simulink model "Coords_Model_1_alt_variation"  (R2019b)
settings: Solver=ode45  StartTime=0.0  StopTime=250  MaxStep=0.02  RelTol=1e-5  AbsTol=1e-7
undefined symbols (not defined in the file): f, ft, m, s
libraries: simulink x6, aerolibutil x2, aerolibconvert2 x2, shared6dof x1, vrlib x1, aerolibconvert x1, dspsnks4 x1, dspvision x1
Description:
  | Six Degree of Freedom Motion Platform
  | 
  | This model shows how to connect an Aerospace Blockset(TM) six degree of freedom
  | equation of motion block.
settings Model: SimulationMode=accelerator  ExtModeTrigMode=oneshot  ExtModeArmWhenConnect=off  ExtModeAutoUpdateStatusClock=off  Creator=The MathWorks, Inc.  LastModifiedBy=Admin
settings SolverCC: AutoScaleAbsTol=off
settings DataIOCC: SaveFormat=Array  SaveOutput=off  ReturnWorkspaceOutputs=off
settings OptimizationCC: DefaultParameterBehavior=Inlined  InlineInvariantSignals=on  ExpressionDepthLimit=2147483647  InitFltsAndDblsToZero=on  EfficientFloat2IntCast=on  LifeSpan=inf
settings DebuggingCC: SaveWithParameterizedLinksMsg=none  MultiTaskCondExecSysMsg=none  SigSpecEnsureSampleTimeMsg=none  FcnCallInpInsideContextMsg=warning  UniqueDataStoreMsg=error  StateNameClashWarn=warning  StrictBusMsg=ErrorOnBusTreatedAsVector  SFUnexpectedBacktrackingDiag=warning  SFNoUnconditionalDefaultTransitionDiag=warning  SFExecutionAtInitializationDiag=none  ArithmeticOperatorsInVariantConditions=warning
settings HardwareCC: ProdBitPerPointer=32  ProdLargestAtomicFloat=None  ProdIntDivRoundTo=Undefined  ProdEndianess=Unspecified  ProdWordSize=32  ProdHWDeviceType=32-bit Generic  TargetUnknown=on
settings ModelReferenceCC: PropagateSignalLabelsOutOfModel=off
settings SFSimCC: SimUseLocalCustomCode=off  CustomCodeUndefinedFunction=UseInterfaceOnly
settings RTWCC: TemplateMakefile=grt_vc.tmf  RTWUseLocalCustomCode=off
settings CodeAppCC: StateflowObjectComments=on
settings GRTTargetCC: TargetFcnLib=ansi_tfl_tmw.mat  TargetLangStandard=C89/C90 (ANSI)  GeneratePreprocessorConditionals=Disable all  CombineOutputUpdateFcns=off  GRTInterface=on
settings ConfigComp: CovMetricSettings=d  CovHtmlReporting=on  CovSaveCumulativeToWorkspaceVar=on  CovSaveSingleToWorkspaceVar=on  CovExternalEMLEnable=off

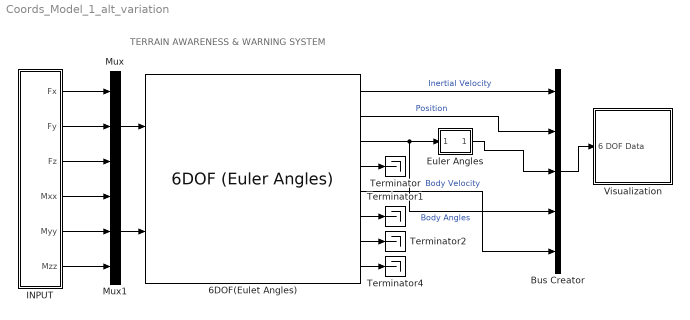
== system Coords_Model_1_alt_variation ==
  note: TERRAIN AWARENESS & WARNING SYSTEM
  "6DOF(Eulet Angles) " : shared6dof/6DOF (Euler Angles)  units=Metric (MKS)  mtype=Fixed  rep=Euler Angles  xme_0=[8500 0 -850]  Vm_0=[0 -75 0]  eul_0=[-0.05 0.1 -0.1]  pm_0=[0 0 0]  mass_0=1.0  mass_e=0.5  mass_f=2.0  inertia=eye(3)  inertia_e=eye(3)  inertia_f=2*eye(3)  k_quat=1.0  vre_flag=on  abi_flag=off  aMode=0  xme_statename=''  Vm_statename=''  eul_statename=''  quat_statename=''  pm_statename=''  mass_statename=''
      settings: SourceProductBaseCode=AE
  Bus Creator : BusCreator  Inputs=5
  Euler Angles : Subsystem
  INPUT : Subsystem
  Mux : Mux  Inputs=3
  Mux1 : Mux  Inputs=3
  Terminator{,1..2,4} (4 alike) : Terminator
  Visualization : Subsystem
  wires:
  Mux1/1 -> "6DOF(Eulet Angles) "/2
  Mux/1 -> "6DOF(Eulet Angles) "/1
  "6DOF(Eulet Angles) "/1 -> Bus Creator/1  "Inertial Velocity"
  "6DOF(Eulet Angles) "/2 -> Bus Creator/2  "Position"
  "6DOF(Eulet Angles) "/3 -> Bus Creator/4, Euler Angles/1(body angles)  "Body Angles"
  "6DOF(Eulet Angles) "/5 -> Bus Creator/5  "Body Velocity"
  Bus Creator/1 -> Visualization/1(6 DOF Data)
  INPUT/1(Fx) -> Mux/1
  INPUT/2(Fy) -> Mux/2
  INPUT/3(Fz) -> Mux/3
  INPUT/4(Mxx) -> Mux1/1
  INPUT/5(Myy) -> Mux1/2
  INPUT/6(Mzz) -> Mux1/3
  Euler Angles/1(euler angles) -> Bus Creator/3
  "6DOF(Eulet Angles) "/4 -> Terminator/1
  "6DOF(Eulet Angles) "/6 -> Terminator1/1
  "6DOF(Eulet Angles) "/7 -> Terminator2/1
  "6DOF(Eulet Angles) "/8 -> Terminator4/1

== system Coords_Model_1_alt_variation/Euler Angles ==
  body angles : Inport
  Bus Creator1 : BusCreator  Inputs=3
  Demux : Demux  Outputs=3
  euler angles : Outport
  wires:
  body angles/1 -> Demux/1
  Bus Creator1/1 -> euler angles/1  "euler angles"
  Demux/1 -> Bus Creator1/1  "psi"
  Demux/2 -> Bus Creator1/2  "theta"
  Demux/3 -> Bus Creator1/3  "phi"

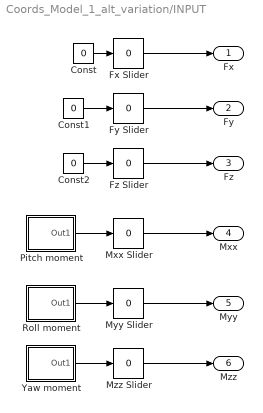
== system Coords_Model_1_alt_variation/INPUT ==
  Const : Constant  Value=0
  Const1 : Constant  Value=0
  Const2 : Constant  Value=0
  Fx Slider : simulink/Math Operations/Slider Gain  gain=0  low=-1  high=1
  Fy Slider : simulink/Math Operations/Slider Gain  gain=0  low=-1  high=1
  Fz Slider : simulink/Math Operations/Slider Gain  gain=0  low=-1  high=1
  Mxx Slider : simulink/Math Operations/Slider Gain  gain=0  low=-5  high=10
  Myy Slider : simulink/Math Operations/Slider Gain  gain=0  low=-10  high=10
  Mzz Slider : simulink/Math Operations/Slider Gain  gain=0  low=-1  high=1
  Pitch moment : Subsystem  mask(timed input){t=[0 3 3 4 4 5 5  7.5 7.5 8.5 8.5 9.5 9.5 10], u=[0 0  1 1 -1 -1.005 0 0 -1 -1 1 1 0 0]*3.138/2}
      mask prompts: t "time values:"; u "input values"
      mask Display: plot(t,u)
  Roll moment : Subsystem  mask(timed input){t=[0 1 1 2 2  10], u=[1 1 -1 -.998  0 0]*3.144/2}
      mask prompts: t "time values:"; u "input values"
      mask Display: plot(t,u)
  Yaw moment : Subsystem  mask(timed input){t=[0 6 6 7 7 8 8 10], u=[0 0  -1 -1 1 1 0 0]*3.1/2}
      mask prompts: t "time values:"; u "input values"
      mask Display: plot(t,u)
  Fx : Outport
  Fy : Outport  Port=2
  Fz : Outport  Port=3
  Mxx : Outport  Port=4
  Myy : Outport  Port=5
  Mzz : Outport  Port=6
  wires:
  Roll moment/1(Out1) -> Myy Slider/1
  Yaw moment/1(Out1) -> Mzz Slider/1
  Const2/1 -> Fz Slider/1
  Const/1 -> Fx Slider/1
  Pitch moment/1(Out1) -> Mxx Slider/1
  Const1/1 -> Fy Slider/1
  Fy Slider/1 -> Fy/1
  Mxx Slider/1 -> Mxx/1
  Myy Slider/1 -> Myy/1
  Fz Slider/1 -> Fz/1
  Fx Slider/1 -> Fx/1
  Mzz Slider/1 -> Mzz/1

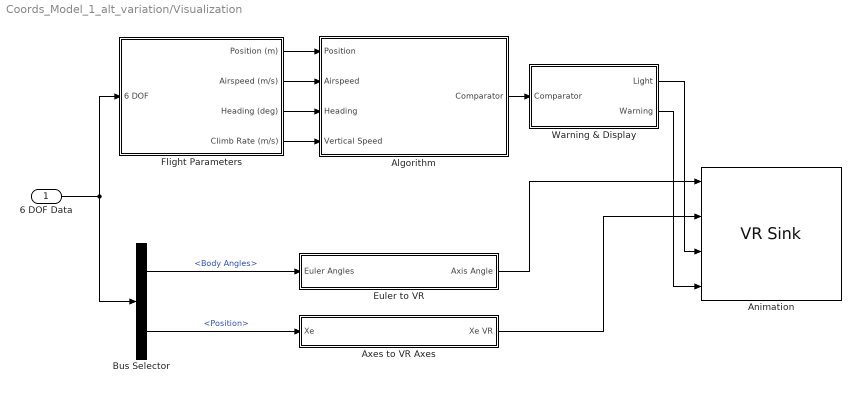
== system Coords_Model_1_alt_variation/Visualization ==
  6 DOF Data : Inport
  Algorithm : Subsystem
  Animation : vrlib/VR Sink  InstantiateOnLoad=on  SampleTime=0.1  ViewEnable=on  RemoteChange=off  RemoteView=off  FieldsWritten=Plane.rotation.4.1.1.double#Plane.translation.3.1.1.double#Light.diffuseColor.3.1.1.double#Warning.string.1.-1.1.char  WorldFileName=Coods_Updated.wrl  WorldDescription=VR Plane Take-Off with HUD Text  AutoView=off  VideoDimensions=[]  AllowVariableSize=off
      settings: SourceProductName=Simulink
  Axes to VR Axes : Subsystem
  Bus Selector : BusSelector  OutputSignals=Body Angles,Position
  Euler to VR : Subsystem
  "Flight Parameters " : Subsystem
  Warning & Display : Subsystem
  wires:
  6 DOF Data/1 -> Bus Selector/1, "Flight Parameters "/1("6 DOF ")
  Bus Selector/2 -> Axes to VR Axes/1(Xe)  "<Position>"
  Bus Selector/1 -> Euler to VR/1(Euler Angles)  "<Body Angles>"
  Algorithm/1(Comparator) -> Warning & Display/1(Comparator)
  "Flight Parameters "/1(Position (m)) -> Algorithm/1(Position)
  "Flight Parameters "/2(Airspeed (m/s)) -> Algorithm/2(Airspeed)
  "Flight Parameters "/3(Heading (deg)) -> Algorithm/3(Heading)
  Warning & Display/1(Light) -> Animation/3
  Warning & Display/2(Warning) -> Animation/4
  Euler to VR/1(Axis Angle) -> Animation/1
  Axes to VR Axes/1(Xe VR) -> Animation/2
  "Flight Parameters "/4(Climb Rate (m/s)) -> Algorithm/4(Vertical Speed)

== system Coords_Model_1_alt_variation/INPUT/Pitch moment ==
  From Workspace : FromWorkspace  VariableName=[t',u']  SampleTime=0
  Out1 : Outport  VectorParamsAs1DForOutWhenUnconnected=off
  wires:
  From Workspace/1 -> Out1/1

== system Coords_Model_1_alt_variation/INPUT/Roll moment ==
  From Workspace : FromWorkspace  VariableName=[t',u']  SampleTime=0
  Out1 : Outport  VectorParamsAs1DForOutWhenUnconnected=off
  wires:
  From Workspace/1 -> Out1/1

== system Coords_Model_1_alt_variation/INPUT/Yaw moment ==
  From Workspace : FromWorkspace  VariableName=[t',u']  SampleTime=0
  Out1 : Outport  VectorParamsAs1DForOutWhenUnconnected=off
  wires:
  From Workspace/1 -> Out1/1

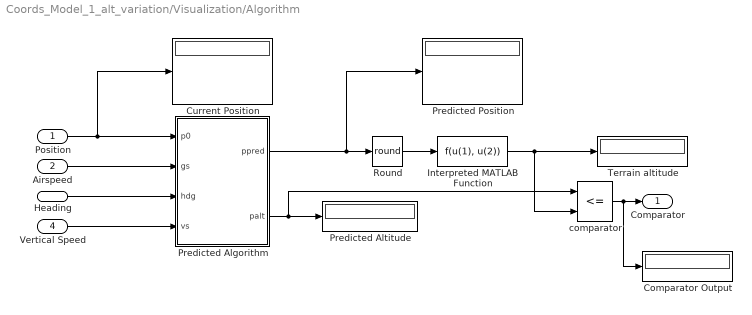
== system Coords_Model_1_alt_variation/Visualization/Algorithm ==
  Position : Inport
  Airspeed : Inport  Port=2
  Heading : Inport  Port=3
  Vertical Speed : Inport  Port=4
  Comparator Output : Display
  Current Position : Display
  Interpreted MATLAB Function : MATLABFcn  MATLABFcn=f(u(1), u(2))
      mask init:
      | load('interpo.mat')
  Predicted Algorithm : MATLAB Function  TreatAsAtomicUnit=on
  Predicted Altitude : Display
      settings: Format=bank
  Predicted Position : Display
  Round : Rounding  Operator=round
  Terrain altitude : Display
  comparator : RelationalOperator  Operator=<=  OutDataTypeStr=boolean  RndMeth=Simplest
  Comparator : Outport
  wires:
  Heading/1 -> Predicted Algorithm/3(hdg)
  Round/1 -> Interpreted MATLAB Function/1
  Interpreted MATLAB Function/1 -> Terrain altitude/1, comparator/2
  Position/1 -> Current Position/1, Predicted Algorithm/1(p0)
  Predicted Algorithm/2(palt) -> Predicted Altitude/1, comparator/1
  Airspeed/1 -> Predicted Algorithm/2(gs)
  comparator/1 -> Comparator Output/1, Comparator/1
  Predicted Algorithm/1(ppred) -> Predicted Position/1, Round/1
  Vertical Speed/1 -> Predicted Algorithm/4(vs)

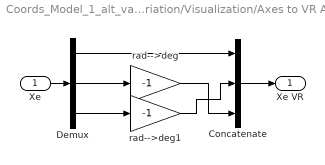
== system Coords_Model_1_alt_variation/Visualization/Axes to VR Axes ==
  Xe : Inport
  Concatenate : Concatenate  NumInputs=3
  Demux : Demux  Outputs=3
  rad-->deg : Gain  Gain=-1  SaturateOnIntegerOverflow=on  OutDataTypeStr=Inherit: Same as input  ParamDataTypeStr=Inherit: Same as input
  rad-->deg1 : Gain  Gain=-1  SaturateOnIntegerOverflow=on  OutDataTypeStr=Inherit: Same as input  ParamDataTypeStr=Inherit: Same as input
  Xe VR : Outport  VectorParamsAs1DForOutWhenUnconnected=off
  wires:
  Xe/1 -> Demux/1
  Demux/1 -> Concatenate/1
  Demux/2 -> rad-->deg/1
  Demux/3 -> rad-->deg1/1
  Concatenate/1 -> Xe VR/1
  rad-->deg1/1 -> Concatenate/2
  rad-->deg/1 -> Concatenate/3

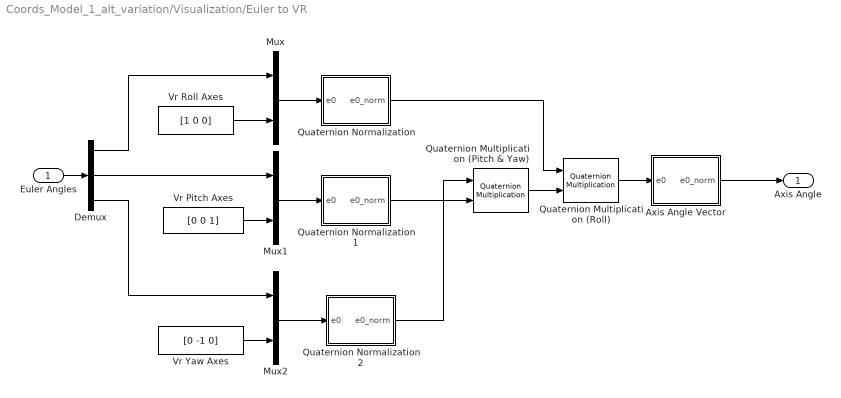
== system Coords_Model_1_alt_variation/Visualization/Euler to VR ==
  Euler Angles : Inport
  Axis Angle Vector : Subsystem
  Demux : Demux  Outputs=3
  Mux : Mux  Inputs=2
  Mux1 : Mux  Inputs=2
  Mux2 : Mux  Inputs=2
  Quaternion Multiplication (Pitch & Yaw) : aerolibutil/Quaternion Multiplication
  Quaternion Multiplication (Roll) : aerolibutil/Quaternion Multiplication
  Quaternion Normalization : Subsystem
  Quaternion Normalization1 : Subsystem
  Quaternion Normalization2 : Subsystem
  Vr Pitch Axes : Constant  Value=[0 0 1]
  Vr Roll Axes : Constant  Value=[1 0 0]
  Vr Yaw Axes : Constant  Value=[0 -1 0]
  Axis Angle : Outport  VectorParamsAs1DForOutWhenUnconnected=off
  wires:
  Quaternion Multiplication (Roll)/1 -> Axis Angle Vector/1(e0)
  Quaternion Multiplication (Pitch & Yaw)/1 -> Quaternion Multiplication (Roll)/2
  Axis Angle Vector/1(e0_norm) -> Axis Angle/1
  Quaternion Normalization/1(e0_norm) -> Quaternion Multiplication (Roll)/1
  Quaternion Normalization2/1(e0_norm) -> Quaternion Multiplication (Pitch & Yaw)/1
  Quaternion Normalization1/1(e0_norm) -> Quaternion Multiplication (Pitch & Yaw)/2
  Mux2/1 -> Quaternion Normalization2/1(e0)
  Mux1/1 -> Quaternion Normalization1/1(e0)
  Mux/1 -> Quaternion Normalization/1(e0)
  Demux/3 -> Mux2/1
  Vr Yaw Axes/1 -> Mux2/2
  Demux/2 -> Mux1/1
  Vr Pitch Axes/1 -> Mux1/2
  Demux/1 -> Mux/1
  Vr Roll Axes/1 -> Mux/2
  Euler Angles/1 -> Demux/1

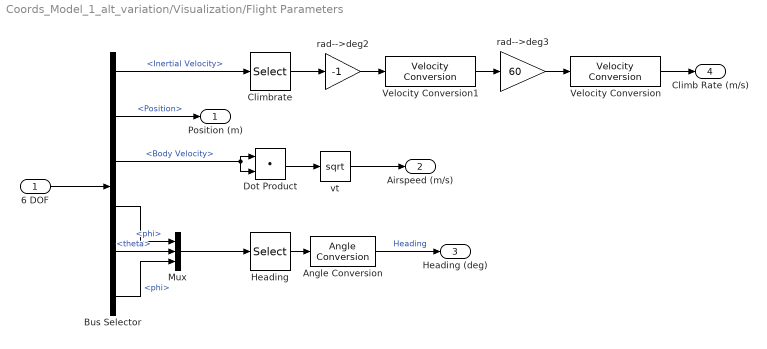
== system Coords_Model_1_alt_variation/Visualization/Flight Parameters  ==
  "6 DOF " : Inport
  Angle Conversion : aerolibconvert2/Angle Conversion  IU=rad  OU=deg
  Bus Selector : BusSelector  OutputSignals=Inertial Velocity,Position,Body Velocity,euler angles.phi,euler angles.theta,euler angles.phi
  Climbrate : Selector  IndexMode=Zero-based  InputPortWidth=3  IndexOptions=Index vector (dialog)  Indices=2  OutputSizes=1
  Dot Product : DotProduct  SaturateOnIntegerOverflow=on  OutDataTypeStr=Inherit: Inherit via internal rule
  Heading : Selector  IndexMode=Zero-based  InputPortWidth=3  IndexOptions=Index vector (dialog)  Indices=2  OutputSizes=1
  Mux : Mux  Inputs=3
  Velocity Conversion : aerolibconvert2/Velocity Conversion  IU=ft/min  OU=m/s
  Velocity Conversion1 : aerolibconvert/Velocity Conversion  IU=m/s  OU=ft/s
      settings: SourceProductName=Aerospace Blockset  SourceProductBaseCode=AE
  rad-->deg2 : Gain  Gain=-1  SaturateOnIntegerOverflow=on  OutDataTypeStr=Inherit: Same as input  ParamDataTypeStr=Inherit: Same as input
  rad-->deg3 : Gain  Gain=60  SaturateOnIntegerOverflow=on  OutDataTypeStr=Inherit: Same as input  ParamDataTypeStr=Inherit: Same as input
  vt : Sqrt  SaturateOnIntegerOverflow=on
  Position (m) : Outport  VectorParamsAs1DForOutWhenUnconnected=off
  Airspeed (m/s) : Outport  Port=2  VectorParamsAs1DForOutWhenUnconnected=off
  Heading (deg) : Outport  Port=3  VectorParamsAs1DForOutWhenUnconnected=off
  Climb Rate (m/s) : Outport  Port=4  VectorParamsAs1DForOutWhenUnconnected=off
  wires:
  Bus Selector/1 -> Climbrate/1  "<Inertial Velocity>"
  Angle Conversion/1 -> Heading (deg)/1  "Heading"
  Heading/1 -> Angle Conversion/1
  Mux/1 -> Heading/1
  vt/1 -> Airspeed (m/s)/1
  Dot Product/1 -> vt/1
  Bus Selector/3 -> Dot Product/2, Dot Product/1  "<Body Velocity>"
  "6 DOF "/1 -> Bus Selector/1
  Bus Selector/4 -> Mux/1  "<phi>"
  Bus Selector/5 -> Mux/2  "<theta>"
  Bus Selector/6 -> Mux/3  "<phi>"
  Bus Selector/2 -> Position (m)/1  "<Position>"
  Climbrate/1 -> rad-->deg2/1
  Velocity Conversion1/1 -> rad-->deg3/1
  rad-->deg2/1 -> Velocity Conversion1/1
  rad-->deg3/1 -> Velocity Conversion/1
  Velocity Conversion/1 -> Climb Rate (m/s)/1

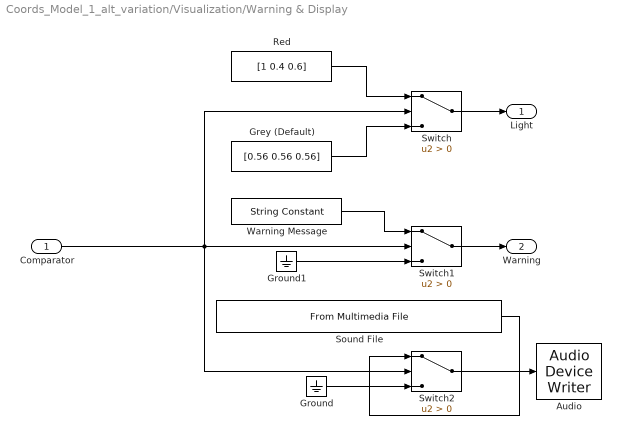
== system Coords_Model_1_alt_variation/Visualization/Warning & Display ==
  Comparator : Inport
  "Audio " : dspsnks4/Audio Device Writer  Driver=DirectSound  Device=Default  InheritSampleRate=on  SampleRate=20  BitDepth=16-bit integer  BufferSize=4096  NumBuffers=10  DefaultOutputChannelMapping=on  OutputChannelMapping=1:2  OutputNumUnderrunSamples=off  DriverIdx=1  DeviceWarnFlag=''
  Grey (Default) : Constant  Value=[0.56 0.56 0.56]
  Ground : Ground
  Ground1 : Ground
  Red : Constant  Value=[1 0.4 0.6]
  Sound File : dspvision/From Multimedia File  inputFilename=D:\B.Tech Thesis\TAWS_Final_Files\BEEP SOUND.mp3  readRange=[1 Inf]  loop=on  numPlays=inf  outputStreams=Audio only  videoDataType=single  audioDataType=double  inheritSampleTime=off  userDefinedSampleTime=1/100  noAudioOutput=off  isIntensityVideo=off  fourcc=RGB  colorVideoFormat=Separate color signals  outputEOF=off  dataOrg=Column-major  audioFrameSize=1024  computeAudioFrameSize=off  outSamplingMode=Sample based
      settings: SourceProductName=DSP System Toolbox  SourceProductBaseCode=DS
  Switch : Switch  Criteria=u2 > Threshold
  Switch1 : Switch  Criteria=u2 > Threshold
  Switch2 : Switch  Criteria=u2 > Threshold
  Warning Message : StringConstant  String="\"TERRAIN...TERRAIN\""
  Light : Outport
  Warning : Outport  Port=2
  wires:
  Ground1/1 -> Switch1/3
  Switch1/1 -> Warning/1
  Red/1 -> Switch/1
  Warning Message/1 -> Switch1/1
  Grey (Default)/1 -> Switch/3
  Switch/1 -> Light/1
  Comparator/1 -> Switch2/2, Switch/2, Switch1/2
  Ground/1 -> Switch2/3
  Sound File/1 -> Switch2/1
  Switch2/1 -> "Audio "/1

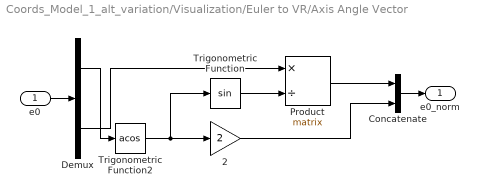
== system Coords_Model_1_alt_variation/Visualization/Euler to VR/Axis Angle Vector ==
  e0 : Inport
  2 : Gain  Gain=2  SaturateOnIntegerOverflow=on  OutDataTypeStr=Inherit: Same as input  ParamDataTypeStr=Inherit: Same as input
  Concatenate : Concatenate
  Demux : Demux  Outputs=[1 3 ]
  Product : Product  Inputs=*/  Multiplication=Matrix(*)  SaturateOnIntegerOverflow=on  InputSameDT=on  OutDataTypeStr=Inherit: Same as first input
  Trigonometric Function : Trigonometry
  Trigonometric Function2 : Trigonometry  Operator=acos
  e0_norm : Outport  VectorParamsAs1DForOutWhenUnconnected=off
  wires:
  Demux/1 -> Trigonometric Function2/1
  Demux/2 -> Product/1
  Concatenate/1 -> e0_norm/1
  Product/1 -> Concatenate/1
  2/1 -> Concatenate/2
  Trigonometric Function/1 -> Product/2
  Trigonometric Function2/1 -> Trigonometric Function/1, 2/1
  e0/1 -> Demux/1

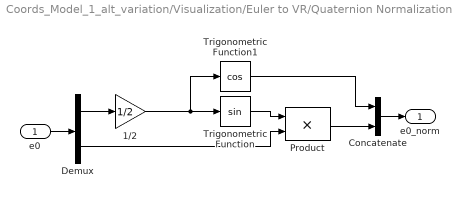
== system Coords_Model_1_alt_variation/Visualization/Euler to VR/Quaternion Normalization ==
  e0 : Inport
  1/2 : Gain  Gain=1/2  SaturateOnIntegerOverflow=on  OutDataTypeStr=Inherit: Same as input  ParamDataTypeStr=Inherit: Same as input
  Concatenate : Concatenate
  Demux : Demux  Outputs=[1 3]
  Product : Product  SaturateOnIntegerOverflow=on  InputSameDT=on  OutDataTypeStr=Inherit: Same as first input
  Trigonometric Function : Trigonometry
  Trigonometric Function1 : Trigonometry  Operator=cos
  e0_norm : Outport  VectorParamsAs1DForOutWhenUnconnected=off
  wires:
  Trigonometric Function1/1 -> Concatenate/1
  Demux/2 -> Product/2
  Demux/1 -> 1/2/1
  Concatenate/1 -> e0_norm/1
  Product/1 -> Concatenate/2
  Trigonometric Function/1 -> Product/1
  1/2/1 -> Trigonometric Function1/1, Trigonometric Function/1
  e0/1 -> Demux/1

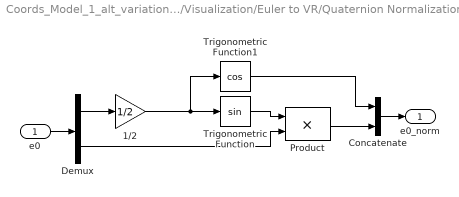
== system Coords_Model_1_alt_variation/Visualization/Euler to VR/Quaternion Normalization1 ==
  e0 : Inport
  1/2 : Gain  Gain=1/2  SaturateOnIntegerOverflow=on  OutDataTypeStr=Inherit: Same as input  ParamDataTypeStr=Inherit: Same as input
  Concatenate : Concatenate
  Demux : Demux  Outputs=[1 3]
  Product : Product  SaturateOnIntegerOverflow=on  InputSameDT=on  OutDataTypeStr=Inherit: Same as first input
  Trigonometric Function : Trigonometry
  Trigonometric Function1 : Trigonometry  Operator=cos
  e0_norm : Outport  VectorParamsAs1DForOutWhenUnconnected=off
  wires:
  e0/1 -> Demux/1
  1/2/1 -> Trigonometric Function/1, Trigonometric Function1/1
  Trigonometric Function/1 -> Product/1
  Product/1 -> Concatenate/2
  Concatenate/1 -> e0_norm/1
  Demux/1 -> 1/2/1
  Demux/2 -> Product/2
  Trigonometric Function1/1 -> Concatenate/1

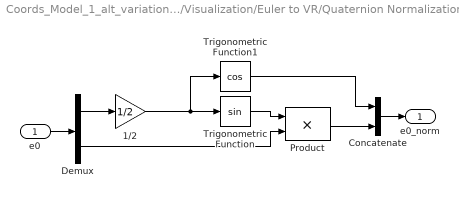
== system Coords_Model_1_alt_variation/Visualization/Euler to VR/Quaternion Normalization2 ==
  e0 : Inport
  1/2 : Gain  Gain=1/2  SaturateOnIntegerOverflow=on  OutDataTypeStr=Inherit: Same as input  ParamDataTypeStr=Inherit: Same as input
  Concatenate : Concatenate
  Demux : Demux  Outputs=[1 3]
  Product : Product  SaturateOnIntegerOverflow=on  InputSameDT=on  OutDataTypeStr=Inherit: Same as first input
  Trigonometric Function : Trigonometry
  Trigonometric Function1 : Trigonometry  Operator=cos
  e0_norm : Outport  VectorParamsAs1DForOutWhenUnconnected=off
  wires:
  Trigonometric Function1/1 -> Concatenate/1
  Demux/2 -> Product/2
  Demux/1 -> 1/2/1
  Concatenate/1 -> e0_norm/1
  Product/1 -> Concatenate/2
  Trigonometric Function/1 -> Product/1
  1/2/1 -> Trigonometric Function1/1, Trigonometric Function/1
  e0/1 -> Demux/1

== matlab function Coords_Model_1_alt_variation/Visualization/Algorithm/Predicted Algorithm ==
  data: p0 input size=[1 3]; gs input; hdg input; ppred output; palt output; vs input
function [ppred, palt] = fcn(p0,gs,hdg,vs)

%Path Prediction
theta = 90-hdg;
v = [-gs*cosd(theta), gs*sind(theta), vs]; 
ppred = p0 - (30*v);
palt = -p0(3) + (vs*30);
